simulink model "BMM_WholeCochlea"  (R2025a)
settings: Solver=VariableStepAuto  StartTime=0.0  StopTime=1  FixedStep=1/48000  RelTol=1e-3
model workspace (MAT data in the model file):
  C_1 = 1e-07
  C_10 = 2.26271743937e-06
  C_11 = 3.19996187844e-06
  C_2 = 1.41421187761e-07
  C_3 = 1.99999523478e-07
  C_4 = 2.8284170162e-07
  C_5 = 3.99998093915e-07
  C_6 = 5.65682055438e-07
  C_7 = 7.99994281752e-07
  C_8 = 1.13136141528e-06
  C_9 = 1.59998475136e-06
  L_0 = 0.033
  L_1 = 0.01
  L_10 = 0.01
  L_11 = 0.01
  L_2 = 0.01
  L_3 = 0.01
  L_4 = 0.01
  L_5 = 0.01
  L_6 = 0.01
  L_7 = 0.01
  L_8 = 0.01
  L_9 = 0.01
  Ls_1 = 0.033
  Ls_10 = 0.033
  Ls_11 = 0.033
  Ls_2 = 0.033
  Ls_3 = 0.033
  Ls_4 = 0.033
  Ls_5 = 0.033
  Ls_6 = 0.033
  Ls_7 = 0.033
  Ls_8 = 0.033
  Ls_9 = 0.033
  R_1 = 150
  R_10 = 31.5337846203
  R_11 = 26.5166622413
  R_2 = 126.13453742
  R_3 = 106.066143535
  R_4 = 89.1906930052
  R_5 = 75.0001786961
  R_6 = 63.0674189752
  R_7 = 53.0331981249
  R_8 = 44.5954527561
  R_9 = 37.5001786963
  U_inputGain = 2
libraries: spsSeriesRLCBranchLib x26, spsGroundLib x15, spsCurrentMeasurementLib x12, spsVoltageMeasurementLib x3, spsControlledVoltageSourceLib x2, simulink x1, sps_lib x1
settings Model: Creator=rsalo  LastModifiedBy=kgl07
settings SolverCC: AlgebraicLoopSolver=TrustRegion
settings DataIOCC: ReturnWorkspaceOutputs=off
settings DebuggingCC: UnconnectedInputMsg=warning  UnconnectedOutputMsg=warning  UnconnectedLineMsg=warning  ArithmeticOperatorsInVariantConditions=warning
settings ModelReferenceCC: EnableRefExpFcnMdlSchedulingChecks=on
settings SFSimCC: SimUseLocalCustomCode=off  CustomCodeUndefinedFunction=UseInterfaceOnly
settings RTWCC: RTWUseLocalCustomCode=off  GPUComputeCapability=3.5  DLArmComputeVersion=19.05

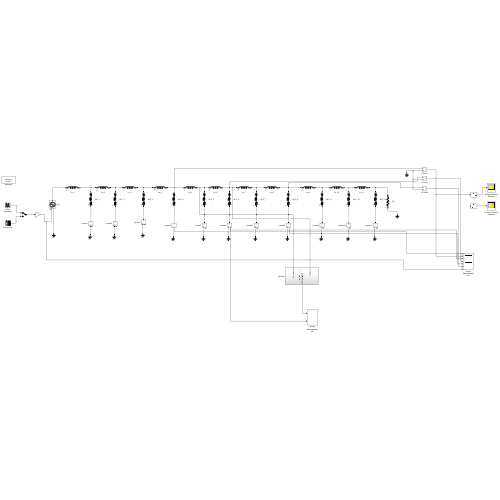
[thumbnail: Simulink's stored preview of the top-level diagram]
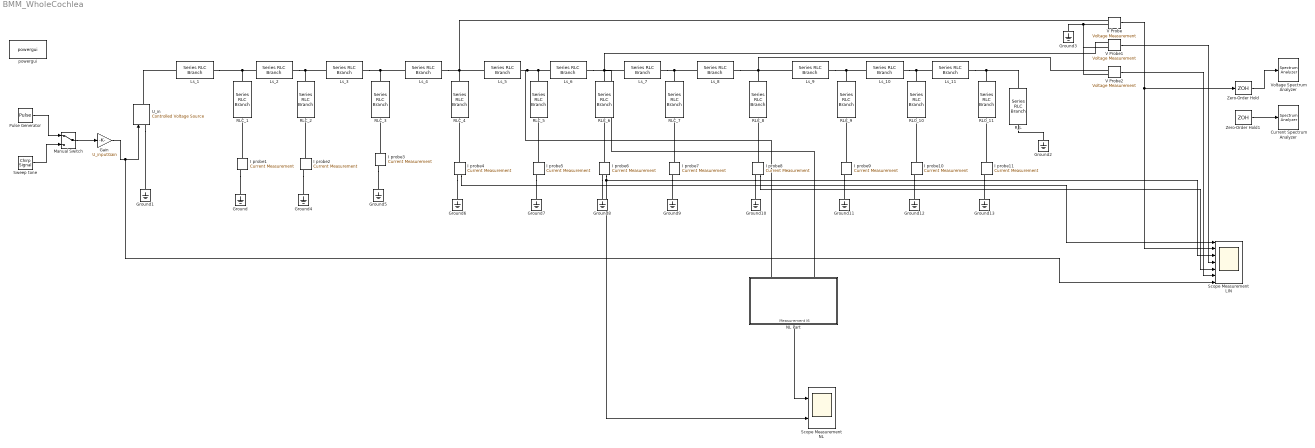
== system BMM_WholeCochlea ==
  Current Spectrum Analyzer : SpectrumAnalyzer  WindowPosition=[107.000000,-33.000000,1309.000000,844.000000,]  Visible=on  ScopeFrameLocation=container  ContainerLayout="{\"WindowBounds\":[99,24,1323,882],\"gridDimensions\":{\"w\":1,\"h\":1},\"tileCount\":1,\"tileCoverage\":1,\"columnWeights\":1,\"rowWeights\":1,\"tileOccupancy\":{\"children\":[{\"id\":\"/Scope\\nMeasurement\\nNL\"},{\"id\":\"/Scope\\nMeasurement\\nLIN\"},{\"id\":\"/Current Spectrum\\nAnalyzer\"},{\"id\":\"/Voltage Spectrum\\nAnalyzer\"}]}}"  Method=Welch  SampleRate=20000  PlotAsTwoSidedSpectrum=off  FrequencyScale=Log  FrequencyResolutionMethod=Window length  WindowLength=2048  FrequencySpan=Start and stop frequencies  StartFrequency=100  StopFrequency=10e3  OverlapPercent=90  AveragingMethod=Running  SpectrumUnits=Watts  PlotNormalTrace=off  PlotMaxHoldTrace=on  YLimits=[-1 1]  AllowFFTLengthLessThanSamplesPerUpdate=on  DefaultConfigurationName=spbscopes.SpectrumAnalyzerBlockCfg  IsFrequencyInputMode=0  FrequencyVectorPort=0  FrequencyVectorFromPort=0  FrequencyInputRBWPort=0  FrequencyInputRBWFromPort=0
  Gain : Gain  Gain=U_inputGain
  Ground{,1..13} (14 alike) : spsGroundLib/Ground  LConnTagsString=a
  I probe{1..11} (11 alike) : spsCurrentMeasurementLib/Current Measurement  PhasorSimulation=off  OutputType=Complex  PSBequivalent=0
  Ls_1 : spsSeriesRLCBranchLib/Series RLC Branch  LConnTagsString=__new0  RConnTagsString=__new0  BranchType=L  Resistance=0  Inductance=Ls_1  SetiL0=off  InitialCurrent=0  Capacitance=0  Setx0=off  InitialVoltage=0  Measurements=None
  Ls_10 : spsSeriesRLCBranchLib/Series RLC Branch  LConnTagsString=__new0  RConnTagsString=__new0  BranchType=L  Resistance=0  Inductance=Ls_10  SetiL0=off  InitialCurrent=0  Capacitance=0  Setx0=off  InitialVoltage=0  Measurements=None
  Ls_11 : spsSeriesRLCBranchLib/Series RLC Branch  LConnTagsString=__new0  RConnTagsString=__new0  BranchType=L  Resistance=0  Inductance=Ls_11  SetiL0=off  InitialCurrent=0  Capacitance=0  Setx0=off  InitialVoltage=0  Measurements=None
  Ls_2 : spsSeriesRLCBranchLib/Series RLC Branch  LConnTagsString=__new0  RConnTagsString=__new0  BranchType=L  Resistance=0  Inductance=Ls_2  SetiL0=off  InitialCurrent=0  Capacitance=0  Setx0=off  InitialVoltage=0  Measurements=None
  Ls_3 : spsSeriesRLCBranchLib/Series RLC Branch  LConnTagsString=__new0  RConnTagsString=__new0  BranchType=L  Resistance=0  Inductance=Ls_3  SetiL0=off  InitialCurrent=0  Capacitance=0  Setx0=off  InitialVoltage=0  Measurements=None
  Ls_4 : spsSeriesRLCBranchLib/Series RLC Branch  LConnTagsString=__new0  RConnTagsString=__new0  BranchType=L  Resistance=0  Inductance=Ls_4  SetiL0=off  InitialCurrent=0  Capacitance=0  Setx0=off  InitialVoltage=0  Measurements=None
  Ls_5 : spsSeriesRLCBranchLib/Series RLC Branch  LConnTagsString=__new0  RConnTagsString=__new0  BranchType=L  Resistance=0  Inductance=Ls_5  SetiL0=off  InitialCurrent=0  Capacitance=0  Setx0=off  InitialVoltage=0  Measurements=None
  Ls_6 : spsSeriesRLCBranchLib/Series RLC Branch  LConnTagsString=__new0  RConnTagsString=__new0  BranchType=L  Resistance=0  Inductance=Ls_5  SetiL0=off  InitialCurrent=0  Capacitance=0  Setx0=off  InitialVoltage=0  Measurements=None
  Ls_7 : spsSeriesRLCBranchLib/Series RLC Branch  LConnTagsString=__new0  RConnTagsString=__new0  BranchType=L  Resistance=0  Inductance=Ls_7  SetiL0=off  InitialCurrent=0  Capacitance=0  Setx0=off  InitialVoltage=0  Measurements=None
  "Ls_8 " : spsSeriesRLCBranchLib/Series RLC Branch  LConnTagsString=__new0  RConnTagsString=__new0  BranchType=L  Resistance=0  Inductance=Ls_8  SetiL0=off  InitialCurrent=0  Capacitance=0  Setx0=off  InitialVoltage=0  Measurements=None
  Ls_9 : spsSeriesRLCBranchLib/Series RLC Branch  LConnTagsString=__new0  RConnTagsString=__new0  BranchType=L  Resistance=0  Inductance=Ls_9  SetiL0=off  InitialCurrent=0  Capacitance=0  Setx0=off  InitialVoltage=0  Measurements=None
  Manual Switch : ManualSwitch
  NL Part : Subsystem
  "Pulse Generator " : DiscretePulseGenerator  PulseType=Time based  Period=1  PulseWidth=0.001  SampleTime=1/48000
  RLC_1 : spsSeriesRLCBranchLib/Series RLC Branch  LConnTagsString=__new0  RConnTagsString=__new0  BranchType=RLC  Resistance=R_1  Inductance=L_1  SetiL0=off  InitialCurrent=0  Capacitance=C_1  Setx0=off  InitialVoltage=0  Measurements=None
  RLC_10 : spsSeriesRLCBranchLib/Series RLC Branch  LConnTagsString=__new0  RConnTagsString=__new0  BranchType=RLC  Resistance=R_10  Inductance=L_10  SetiL0=off  InitialCurrent=0  Capacitance=C_10  Setx0=off  InitialVoltage=0  Measurements=None
  RLC_11 : spsSeriesRLCBranchLib/Series RLC Branch  LConnTagsString=__new0  RConnTagsString=__new0  BranchType=RLC  Resistance=R_11  Inductance=L_11  SetiL0=off  InitialCurrent=0  Capacitance=C_11  Setx0=off  InitialVoltage=0  Measurements=None
  RLC_2 : spsSeriesRLCBranchLib/Series RLC Branch  LConnTagsString=__new0  RConnTagsString=__new0  BranchType=RLC  Resistance=R_2  Inductance=L_2  SetiL0=off  InitialCurrent=0  Capacitance=C_2  Setx0=off  InitialVoltage=0  Measurements=None
  RLC_3 : spsSeriesRLCBranchLib/Series RLC Branch  LConnTagsString=__new0  RConnTagsString=__new0  BranchType=RLC  Resistance=R_3  Inductance=L_3  SetiL0=off  InitialCurrent=0  Capacitance=C_3  Setx0=off  InitialVoltage=0  Measurements=None
  RLC_4 : spsSeriesRLCBranchLib/Series RLC Branch  LConnTagsString=__new0  RConnTagsString=__new0  BranchType=RLC  Resistance=R_4  Inductance=L_4  SetiL0=off  InitialCurrent=0  Capacitance=C_4  Setx0=off  InitialVoltage=0  Measurements=None
  RLC_5 : spsSeriesRLCBranchLib/Series RLC Branch  LConnTagsString=__new0  RConnTagsString=__new0  BranchType=RLC  Resistance=R_5  Inductance=L_5  SetiL0=off  InitialCurrent=0  Capacitance=C_5  Setx0=off  InitialVoltage=0  Measurements=None
  RLC_6 : spsSeriesRLCBranchLib/Series RLC Branch  LConnTagsString=__new0  RConnTagsString=__new0  BranchType=RLC  Resistance=R_6  Inductance=L_6  SetiL0=off  InitialCurrent=0  Capacitance=C_6  Setx0=off  InitialVoltage=0  Measurements=None
  RLC_7 : spsSeriesRLCBranchLib/Series RLC Branch  LConnTagsString=__new0  RConnTagsString=__new0  BranchType=RLC  Resistance=R_7  Inductance=L_7  SetiL0=off  InitialCurrent=0  Capacitance=C_7  Setx0=off  InitialVoltage=0  Measurements=None
  RLC_8 : spsSeriesRLCBranchLib/Series RLC Branch  LConnTagsString=__new0  RConnTagsString=__new0  BranchType=RLC  Resistance=R_8  Inductance=L_8  SetiL0=off  InitialCurrent=0  Capacitance=C_8  Setx0=off  InitialVoltage=0  Measurements=None
  RLC_9 : spsSeriesRLCBranchLib/Series RLC Branch  LConnTagsString=__new0  RConnTagsString=__new0  BranchType=RLC  Resistance=R_9  Inductance=L_9  SetiL0=off  InitialCurrent=0  Capacitance=C_9  Setx0=off  InitialVoltage=0  Measurements=None
  R_L : spsSeriesRLCBranchLib/Series RLC Branch  LConnTagsString=__new0  RConnTagsString=__new0  BranchType=R  Resistance=100  Inductance=1e-3  SetiL0=off  InitialCurrent=0  Capacitance=1e-6  Setx0=off  InitialVoltage=0  Measurements=None
  Scope Measurement LIN : Scope  NumInputPorts=7
      settings: TimeUnits=Metric (based on Time Span)  ActiveDisplayString=3  ActiveDisplayYMinimum=-0.00771  ActiveDisplayYMaximum=0.0077  YLabel=Amplitude  DataLoggingVariableName=Scope_Measurement_LIN
  Scope Measurement NL : Scope  NumInputPorts=2
      settings: TimeUnits=Metric (based on Time Span)  ActiveDisplayYMinimum=-4.9E-5  ActiveDisplayYMaximum=4.5E-5  YLabel=Amplitude  DataLoggingVariableName=Scope_Measurement_NL
  Sweep tone : simulink/Sources/Chirp Signal  f1=20  T=1  f2=10000
  U_in : spsControlledVoltageSourceLib/Controlled Voltage Source  Initialize=on  Source_Type=AC  Amplitude=0  Phase=0  Frequency=0  Measurements=None
  V Probe : spsVoltageMeasurementLib/Voltage Measurement  PhasorSimulation=off  OutputType=Complex  PSBequivalent=0
  V Probe1 : spsVoltageMeasurementLib/Voltage Measurement  PhasorSimulation=off  OutputType=Complex  PSBequivalent=0
  V Probe2 : spsVoltageMeasurementLib/Voltage Measurement  PhasorSimulation=off  OutputType=Complex  PSBequivalent=0
  Voltage Spectrum Analyzer : SpectrumAnalyzer  WindowPosition=[107.000000,-33.000000,1309.000000,844.000000,]  Visible=on  ScopeFrameLocation=container  ContainerLayout="{\"WindowBounds\":[99,24,1323,882],\"gridDimensions\":{\"w\":1,\"h\":1},\"tileCount\":1,\"tileCoverage\":1,\"columnWeights\":1,\"rowWeights\":1,\"tileOccupancy\":{\"children\":[{\"id\":\"/Scope\\nMeasurement\\nNL\"},{\"id\":\"/Scope\\nMeasurement\\nLIN\"},{\"id\":\"/Current Spectrum\\nAnalyzer\"},{\"id\":\"/Voltage Spectrum\\nAnalyzer\"}]}}"  Method=Welch  SampleRate=20000  PlotAsTwoSidedSpectrum=off  FrequencyScale=Log  FrequencyResolutionMethod=Window length  WindowLength=2048  FrequencySpan=Start and stop frequencies  StartFrequency=100  StopFrequency=10e3  OverlapPercent=90  AveragingMethod=Running  SpectrumUnits=Watts  PlotNormalTrace=off  PlotMaxHoldTrace=on  YLimits=[-9.2832e-7 0.00000835487]  AllowFFTLengthLessThanSamplesPerUpdate=on  DefaultConfigurationName=spbscopes.SpectrumAnalyzerBlockCfg  IsFrequencyInputMode=0  FrequencyVectorPort=0  FrequencyVectorFromPort=0  FrequencyInputRBWPort=0  FrequencyInputRBWFromPort=0
  Zero-Order Hold : ZeroOrderHold  SampleTime=-1
  Zero-Order Hold1 : ZeroOrderHold  SampleTime=-1
  powergui : sps_lib/powergui  Priority=1  SimulationMode=Discrete  SampleTime=50e-6  frequency=60  Iterations=50  frequencyindice=0  Pbase=100e6  ErrMax=1e-4  UnitsV=kV  UnitsW=MW  buscounter=0  FunctionMessages=off  echomessages=off  EnableUseOfTLC=off  CurrentSourceSwitches=off  DisableSnubberDevices=off  DisableRonSwitches=off  DisableVfSwitches=off  DisplayEquations=off  AutomaticDiscreteSolvers=off  SolverType=Tustin/Backward Euler (TBE)  Interpol=off  ExternalGateDelay=off  methode=off  Ts=100  x0status=blocks  SPID=off  SwTol=0  HookPort=off  NonlinearTolerance=1e-4  nMaxIteration=100  ContinueOnMaxIteration=off  RestoreLinks=warning  ResistiveCurrentMeasurement=off  Frange=[0:2:500]  Ylog=off  Xlog=on  ShowGrid=off  save=off  variable=ZData  structure=0  ZoomFFT=off  StartTime=0.0  cycles=1  DisplayStyle=1  fundamental=60  FreqAxis=off  MaxFrequency=1000  frequencyindicesteady=1  RmsSteady=1  display=off
  wires:
  Manual Switch/1 -> Gain/1
  Gain/1 -> Scope Measurement LIN/7, U_in/1
  V Probe/1 -> Scope Measurement LIN/2, Zero-Order Hold/1
  Sweep tone/1 -> Manual Switch/2
  "Pulse Generator "/1 -> Manual Switch/1
  Zero-Order Hold/1 -> Voltage Spectrum Analyzer/1
  Zero-Order Hold1/1 -> Current Spectrum Analyzer/1
  NL Part/1("Measurement I6 ") -> Scope Measurement NL/1
  V Probe1/1 -> Scope Measurement LIN/4
  V Probe2/1 -> Scope Measurement LIN/6
  I probe4/1 -> Scope Measurement LIN/1
  I probe6/1 -> Scope Measurement LIN/3, Scope Measurement NL/2
  I probe8/1 -> Scope Measurement LIN/5
  connections:
  U_in/RConn1 -- Ls_1/LConn1
  I probe1/RConn1 -- Ground/LConn1
  I probe1/LConn1 -- RLC_1/LConn1
  U_in/LConn1 -- Ground1/LConn1
  Ground3/LConn1 -- V Probe/LConn2 -- V Probe2/LConn2 -- V Probe1/LConn2
  Ls_1/RConn1 -- RLC_1/RConn1 -- Ls_2/LConn1
  Ls_11/RConn1 -- RLC_11/RConn1 -- R_L/RConn1
  R_L/LConn1 -- Ground2/LConn1
  Ls_2/RConn1 -- Ls_3/LConn1 -- RLC_2/RConn1
  I probe2/LConn1 -- RLC_2/LConn1
  I probe2/RConn1 -- Ground4/LConn1
  Ls_3/RConn1 -- Ls_4/LConn1 -- RLC_3/RConn1
  I probe3/LConn1 -- RLC_3/LConn1
  I probe3/RConn1 -- Ground5/LConn1
  Ls_4/RConn1 -- RLC_4/RConn1 -- V Probe/LConn1 -- Ls_5/LConn1
  I probe4/LConn1 -- RLC_4/LConn1
  I probe4/RConn1 -- Ground6/LConn1
  I probe5/LConn1 -- RLC_5/LConn1
  I probe5/RConn1 -- Ground7/LConn1
  Ls_7/RConn1 -- "Ls_8 "/LConn1 -- RLC_7/RConn1
  I probe7/LConn1 -- RLC_7/LConn1
  I probe7/RConn1 -- Ground9/LConn1
  I probe8/RConn1 -- Ground10/LConn1
  I probe8/LConn1 -- RLC_8/LConn1
  Ls_9/RConn1 -- Ls_10/LConn1 -- RLC_9/RConn1
  I probe9/RConn1 -- Ground11/LConn1
  I probe9/LConn1 -- RLC_9/LConn1
  Ls_10/RConn1 -- Ls_11/LConn1 -- RLC_10/RConn1
  I probe10/RConn1 -- Ground12/LConn1
  I probe10/LConn1 -- RLC_10/LConn1
  I probe11/RConn1 -- Ground13/LConn1
  I probe11/LConn1 -- RLC_11/LConn1
  Ls_5/RConn1 -- Ls_6/LConn1 -- RLC_5/RConn1 -- NL Part/LConn1
  RLC_8/RConn1 -- Ls_9/LConn1 -- V Probe2/LConn1 -- "Ls_8 "/RConn1
  I probe6/LConn1 -- RLC_6/LConn1
  I probe6/RConn1 -- Ground8/LConn1
  Ls_6/RConn1 -- NL Part/LConn2 -- Ls_7/LConn1 -- V Probe1/LConn1 -- RLC_6/RConn1

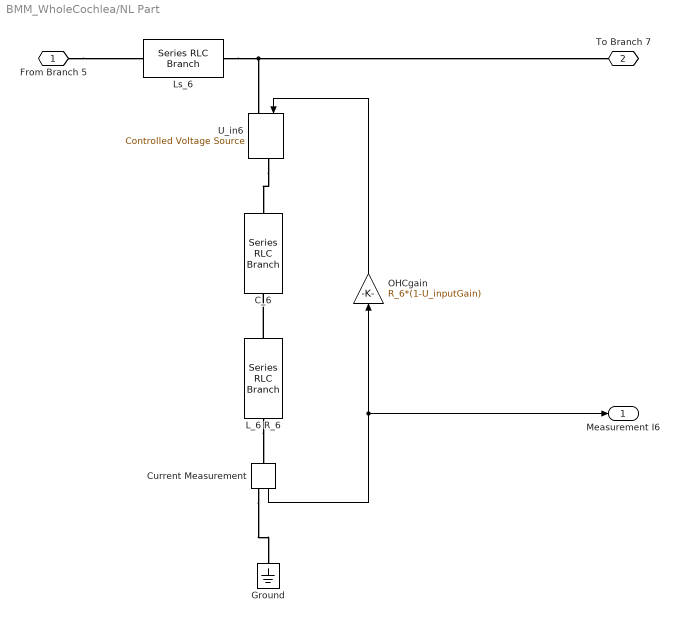
== system BMM_WholeCochlea/NL Part ==
  C_6 : spsSeriesRLCBranchLib/Series RLC Branch  LConnTagsString=__new0  RConnTagsString=__new0  BranchType=C  Resistance=150  Inductance=10e-3  SetiL0=off  InitialCurrent=0  Capacitance=C_6  Setx0=off  InitialVoltage=0  Measurements=None
  Current Measurement : spsCurrentMeasurementLib/Current Measurement  PhasorSimulation=off  OutputType=Complex  PSBequivalent=0
  Ground : spsGroundLib/Ground  LConnTagsString=a
  L_6 R_6 : spsSeriesRLCBranchLib/Series RLC Branch  LConnTagsString=__new0  RConnTagsString=__new0  BranchType=RL  Resistance=R_6  Inductance=L_6  SetiL0=off  InitialCurrent=0  Capacitance=1e-6  Setx0=off  InitialVoltage=0  Measurements=None
  Ls_6 : spsSeriesRLCBranchLib/Series RLC Branch  LConnTagsString=__new0  RConnTagsString=__new0  BranchType=L  Resistance=0  Inductance=Ls_6  SetiL0=off  InitialCurrent=0  Capacitance=0  Setx0=off  InitialVoltage=0  Measurements=None
  OHCgain : Gain  Gain=R_6*(1-U_inputGain)
  U_in6 : spsControlledVoltageSourceLib/Controlled Voltage Source  Initialize=on  Source_Type=AC  Amplitude=0  Phase=0  Frequency=0  Measurements=None
  From Branch 5 : PMIOPort  Side=Left
  To Branch 7 : PMIOPort  Port=2  Side=Left
  "Measurement I6 " : Outport  VectorParamsAs1DForOutWhenUnconnected=off
  wires:
  Current Measurement/1 -> "Measurement I6 "/1, OHCgain/1
  OHCgain/1 -> U_in6/1
  connections:
  Ls_6/RConn1 -- U_in6/LConn1 -- To Branch 7/RConn1
  U_in6/RConn1 -- C_6/RConn1
  From Branch 5/RConn1 -- Ls_6/LConn1
  L_6 R_6/LConn1 -- Current Measurement/LConn1
  Current Measurement/RConn1 -- Ground/LConn1
  L_6 R_6/RConn1 -- C_6/LConn1
